simulink model "s7_template"  (R2023a)
settings: Solver=ode4  StartTime=0.0  StopTime=inf  FixedStep=P_sim_dt  RelTol=1e-3
InitFcn:
  | s6_data;
values from neighbouring files (symbols this model uses):
  P_cx_k = 1    [s6_data.m]
  P_p_Bf = 0.7    [p_mad_car.m]
  P_p_Br = 0.7    [p_mad_car.m]
  P_p_Cf = 2    [p_mad_car.m]
  P_p_Cr = 2    [p_mad_car.m]
  P_p_delta_max = 21.58/180*pi    (= 0.37664205258)    [p_mad_car.m]
  P_p_Df = 2    [p_mad_car.m]
  P_p_Dr = 2.5    [p_mad_car.m]
  P_p_Ef = -0.1    [p_mad_car.m]
  P_p_Er = -0.05    [p_mad_car.m]
  P_p_J = 192e-6    (= 0.000192)    [p_mad_car.m]
  P_p_k = 2.51    [p_mad_car.m]
  P_p_kr = 0.344014    [s6_data.m]
  P_p_l = abs(P_p_frontaxle_1 + P_p_rearaxle_1)    [p_mad_car.m]
  P_p_lf = P_p_frontaxle_1    (= 0.05)    [p_mad_car.m]
  P_p_lr = P_p_rearaxle_1    (= 0.049)    [p_mad_car.m]
  P_p_m = 132e-3    (= 0.132)    [p_mad_car.m]
  P_p_T = 316e-3    (= 0.316)    [p_mad_car.m]
  P_p_TA = 0.02    [s6_data.m]
  P_p_Ti = 0.246830    (= 0.24683)    [s6_data.m]
  P_p_Tt = P_p_uTt + P_p_output_Tt    (= 0.1)    [p_mad_car.m]
undefined symbols (not defined in the file or in its folder): DiscIntNeverNeededParam, Display, mad_lib_template, mbc_car_display
settings Model: Creator=hmekiedj  LastModifiedBy=aaron
settings SolverCC: AlgebraicLoopSolver=TrustRegion
settings DataIOCC: ReturnWorkspaceOutputs=off
settings OptimizationCC: BlockReduction=off  DefaultParameterBehavior=Inlined  BufferReuse=off
settings DebuggingCC: SignalInfNanChecking=warning  UnconnectedInputMsg=warning  UnconnectedOutputMsg=warning  UnconnectedLineMsg=warning  ArithmeticOperatorsInVariantConditions=warning
settings ModelReferenceCC: EnableRefExpFcnMdlSchedulingChecks=on
settings SFSimCC: SimUseLocalCustomCode=off  CustomCodeUndefinedFunction=UseInterfaceOnly
settings RTWCC: RTWUseLocalCustomCode=off
settings CodeAppCC: StateflowObjectComments=on

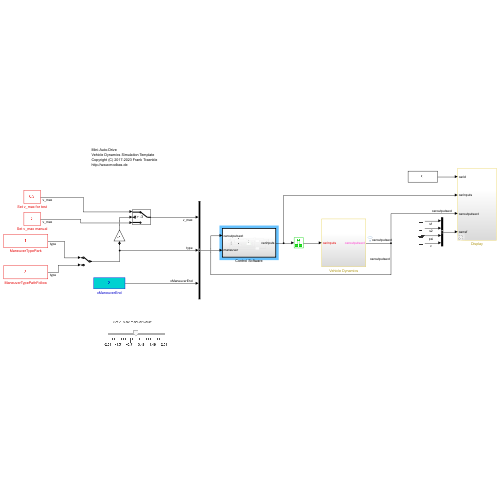
[thumbnail: Simulink's stored preview of the top-level diagram]
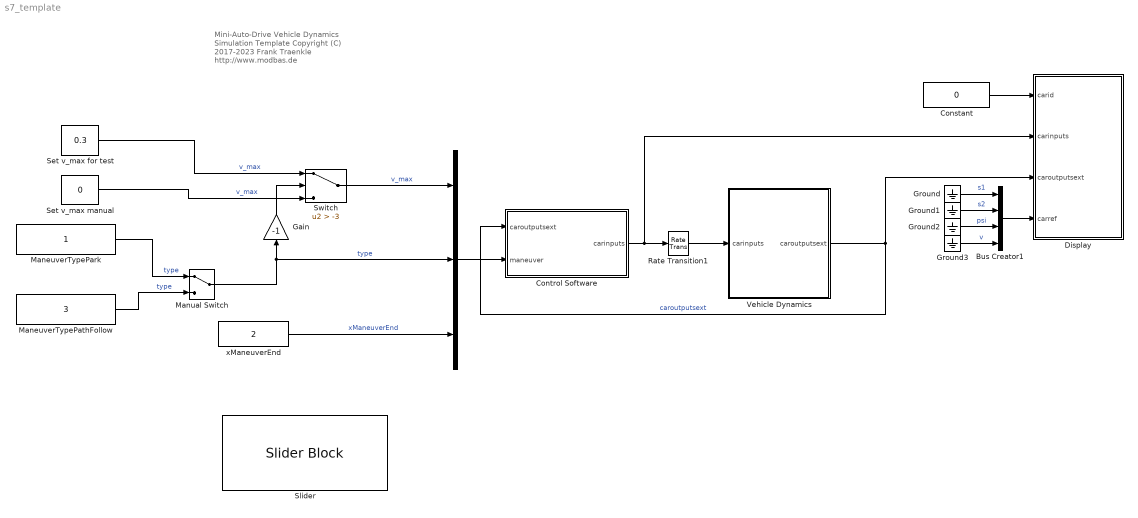
== system s7_template ==
  note: Mini-Auto-Drive
      | Vehicle Dynamics Simulation Template
      | Copyright (C) 2017-2023 Frank Traenkle
      | http://www.modbas.de
  " " : BusCreator  Inputs=3
  Bus Creator1 : BusCreator  Inputs=4
  Constant : Constant  Value=0
  Control Software : Subsystem  TreatAsAtomicUnit=on  SystemSampleTime=P_p_TA
  Display : Subsystem  AncestorBlock=mad_lib_template/Display
      settings: LibrarySourceBlock=mad_lib_template/Display
  Gain : Gain  Gain=-1
  Ground{,1..3} (4 alike) : Ground
  ManeuverTypePark : Constant  SampleTime=-1
  ManeuverTypePathFollow : Constant  Value=3  SampleTime=-1
  Manual Switch : ManualSwitch
  Rate Transition1 : RateTransition
  Set v_max for test : Constant  Value=0.3  SampleTime=-1
  Set v_max manual : Constant  Value=0  SampleTime=-1
  Slider : SliderBlock  ScaleMin=-2.51  ScaleMax=2.51
  Switch : Switch  Criteria=u2 > Threshold  Threshold=-3  SaturateOnIntegerOverflow=off  InputSameDT=off
  Vehicle Dynamics : Subsystem
  xManeuverEnd : Constant  Value=2
  wires:
  Bus Creator1/1 -> Display/4(carref)
  Ground/1 -> Bus Creator1/1  "s1"
  Ground1/1 -> Bus Creator1/2  "s2"
  Ground2/1 -> Bus Creator1/3  "psi"
  Ground3/1 -> Bus Creator1/4  "v"
  Vehicle Dynamics/1(caroutputsext) -> Display/3(caroutputsext), Control Software/1(caroutputsext)  "caroutputsext"
  Rate Transition1/1 -> Vehicle Dynamics/1(carinputs)
  Constant/1 -> Display/1(carid)
  Control Software/1(carinputs) -> Display/2(carinputs), Rate Transition1/1
  " "/1 -> Control Software/2(maneuver)
  xManeuverEnd/1 -> " "/3  "xManeuverEnd"
  ManeuverTypePathFollow/1 -> Manual Switch/2  "type"
  ManeuverTypePark/1 -> Manual Switch/1  "type"
  Manual Switch/1 -> " "/2, Gain/1  "type"
  Switch/1 -> " "/1  "v_max"
  Gain/1 -> Switch/2
  Set v_max for test/1 -> Switch/1  "v_max"
  Set v_max manual/1 -> Switch/3  "v_max"

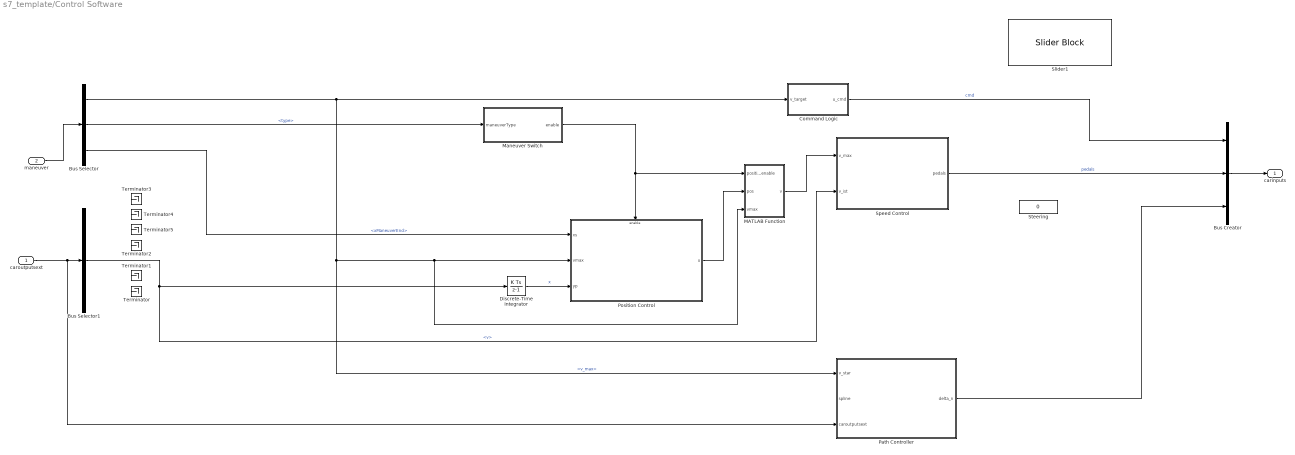
== system s7_template/Control Software ==
  caroutputsext : Inport
  maneuver : Inport  Port=2
  Bus Creator : BusCreator  Inputs=3
  Bus Selector : BusSelector  OutputSignals=v_max,type,xManeuverEnd
  Bus Selector1 : BusSelector  OutputSignals=v
  Command Logic : MATLAB Function  TreatAsAtomicUnit=on
  Discrete-Time Integrator : DiscreteIntegrator  SampleTime=-1  ICPrevOutput=DiscIntNeverNeededParam  ICPrevScaledInput=DiscIntNeverNeededParam
  MATLAB Function : MATLAB Function  TreatAsAtomicUnit=on
  Maneuver Switch : MATLAB Function  TreatAsAtomicUnit=on
  Path Controller : Subsystem
  Position Control : Subsystem
  Slider1 : SliderBlock  LabelPosition=Bottom  ScaleMin=-1  ScaleMax=1
  Speed Control : Subsystem
  Steering : Constant  Value=0  SampleTime=-1
  Terminator{,1..5} (6 alike) : Terminator
  carinputs : Outport
  wires:
  maneuver/1 -> Bus Selector/1
  caroutputsext/1 -> Path Controller/3(caroutputsext), Bus Selector1/1
  Bus Selector1/1 -> Speed Control/2(v_ist), Discrete-Time Integrator/1  "<v>"
  ? -> Terminator/1
  ? -> Terminator1/1
  ? -> Terminator2/1
  ? -> Terminator5/1
  ? -> Terminator4/1
  ? -> Terminator3/1
  Bus Creator/1 -> carinputs/1
  Command Logic/1(u_cmd) -> Bus Creator/1  "cmd"
  Speed Control/1(pedals) -> Bus Creator/2  "pedals"
  Bus Selector/1 -> Path Controller/1(v_star), Position Control/2(vmax), MATLAB Function/3(vmax), Command Logic/1(v_target)  "<v_max>"
  Discrete-Time Integrator/1 -> Position Control/3(yp)  "x"
  Bus Selector/2 -> Maneuver Switch/1(maneuverType)  "<type>"
  Bus Selector/3 -> Position Control/1(xs)  "<xManeuverEnd>"
  Position Control/1(u) -> MATLAB Function/2(pos)
  MATLAB Function/1(v) -> Speed Control/1(v_max)
  Maneuver Switch/1(enable) -> MATLAB Function/1(position_enable), Position Control/Enable
  Path Controller/1(delta_n) -> Bus Creator/3

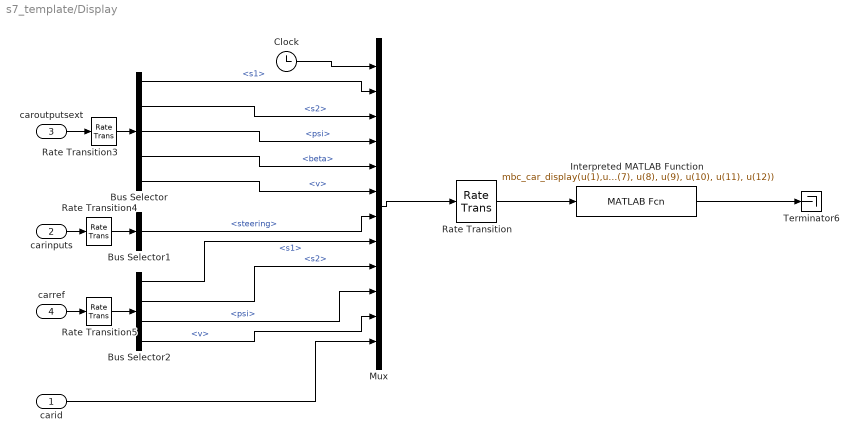
== system s7_template/Display ==
  carid : Inport
  carinputs : Inport  Port=2
  caroutputsext : Inport  Port=3
  carref : Inport  Port=4
  Bus Selector : BusSelector  OutputSignals=s1,s2,psi,beta,v
  Bus Selector1 : BusSelector  OutputSignals=steering
  Bus Selector2 : BusSelector  OutputSignals=s1,s2,psi,v
  Clock : Clock
  Interpreted MATLAB Function : MATLABFcn  MATLABFcn=mbc_car_display(u(1),u(2),u(3),u(4),u(5), u(6), u(7), u(8), u(9), u(10), u(11), u(12))
  Mux : Mux  Inputs=12
  Rate Transition : RateTransition  OutPortSampleTime=P_display_dt
  Rate Transition3 : RateTransition
  Rate Transition4 : RateTransition
  Rate Transition5 : RateTransition
  Terminator6 : Terminator
  wires:
  caroutputsext/1 -> Rate Transition3/1
  Interpreted MATLAB Function/1 -> Terminator6/1
  Mux/1 -> Rate Transition/1
  Rate Transition/1 -> Interpreted MATLAB Function/1
  Clock/1 -> Mux/1
  Bus Selector/1 -> Mux/2  "<s1>"
  Bus Selector/2 -> Mux/3  "<s2>"
  Bus Selector/3 -> Mux/4  "<psi>"
  carinputs/1 -> Rate Transition4/1
  Bus Selector1/1 -> Mux/7  "<steering>"
  Bus Selector/4 -> Mux/5  "<beta>"
  Bus Selector/5 -> Mux/6  "<v>"
  carref/1 -> Rate Transition5/1
  Bus Selector2/4 -> Mux/11  "<v>"
  Bus Selector2/3 -> Mux/10  "<psi>"
  Bus Selector2/2 -> Mux/9  "<s2>"
  Bus Selector2/1 -> Mux/8  "<s1>"
  carid/1 -> Mux/12
  Rate Transition4/1 -> Bus Selector1/1
  Rate Transition3/1 -> Bus Selector/1
  Rate Transition5/1 -> Bus Selector2/1

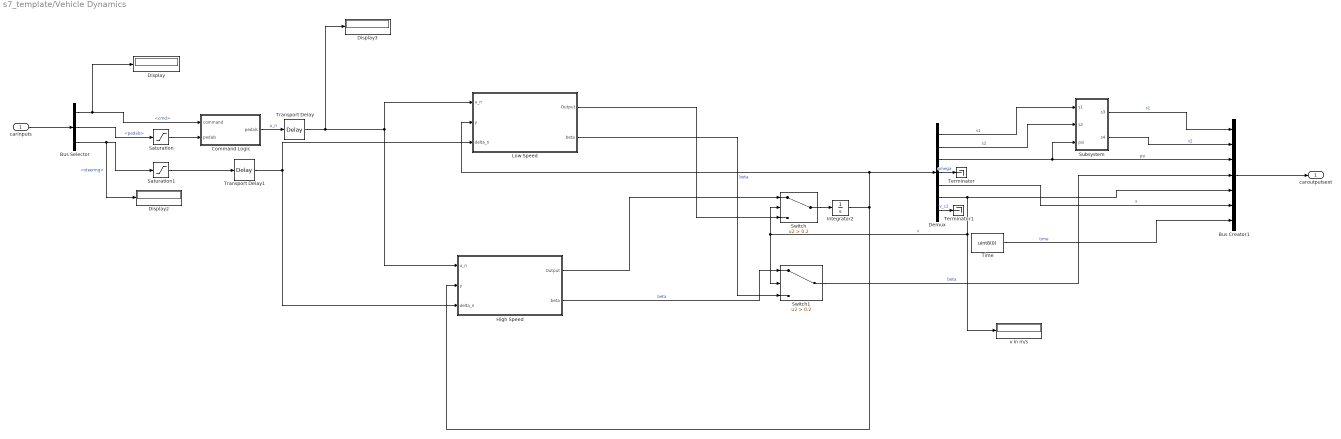
== system s7_template/Vehicle Dynamics ==
  carinputs : Inport
  Bus Creator1 : BusCreator  Inputs=7  OutDataTypeStr=Bus: CAROUTPUTSEXT
  Bus Selector : BusSelector  OutputSignals=cmd,pedals,steering
  Command Logic : MATLAB Function  TreatAsAtomicUnit=on
  Demux : Demux  Outputs=7
  Display : Display
  Display2 : Display
  Display3 : Display
  High Speed : Subsystem
  Integrator2 : Integrator
  Low Speed : Subsystem
  Saturation : Saturate  UpperLimit=1  LowerLimit=-1
  Saturation1 : Saturate  UpperLimit=1  LowerLimit=-1
  Subsystem : Subsystem
  Switch : Switch  Criteria=u2 > Threshold  Threshold=0.2  SaturateOnIntegerOverflow=off  InputSameDT=off
  Switch1 : Switch  Criteria=u2 > Threshold  Threshold=0.2  SaturateOnIntegerOverflow=off  InputSameDT=off
  Terminator : Terminator
  Terminator1 : Terminator
  Time : Constant  Value=uint8(0)
  Transport Delay : TransportDelay  DelayTime=P_p_Tt
  Transport Delay1 : TransportDelay  DelayTime=P_p_Tt
  v in m/s : Display
  caroutputsext : Outport  VectorParamsAs1DForOutWhenUnconnected=off
  wires:
  carinputs/1 -> Bus Selector/1
  Bus Selector/2 -> Saturation/1  "<pedals>"
  Bus Selector/3 -> Saturation1/1, Display2/1  "<steering>"
  Demux/3 -> Subsystem/3(psi), Bus Creator1/3  "psi"
  Bus Creator1/1 -> caroutputsext/1
  Demux/6 -> Switch1/2, Switch/2, v in m/s/1, Bus Creator1/5  "v"
  Time/1 -> Bus Creator1/7  "time"
  Bus Selector/1 -> Display/1, Command Logic/1(command)  "<cmd>"
  Saturation/1 -> Command Logic/2("pedals ")
  Command Logic/1(pedals) -> Transport Delay/1  "u_n"
  Switch/1 -> Integrator2/1
  Transport Delay/1 -> High Speed/1(u_n), Low Speed/1(u_n), Display3/1
  Saturation1/1 -> Transport Delay1/1
  Low Speed/1(Output) -> Switch/3
  Low Speed/2(beta) -> Switch1/3  "beta"
  Switch1/1 -> Bus Creator1/4  "beta"
  Demux/4 -> Terminator/1  "omega"
  High Speed/1(Output) -> Switch/1
  Demux/7 -> Terminator1/1  "v_c2"
  Integrator2/1 -> High Speed/2(y), Low Speed/2(y), Demux/1
  Transport Delay1/1 -> High Speed/3(delta_n), Low Speed/3(delta_n)
  Demux/1 -> Subsystem/1(s1)  "s1"
  Demux/2 -> Subsystem/2(s2)  "s2"
  Subsystem/1(s3) -> Bus Creator1/1  "s1"
  Subsystem/2(s4) -> Bus Creator1/2  "s2"
  Demux/5 -> Bus Creator1/6  "x"
  High Speed/2(beta) -> Switch1/1  "beta"

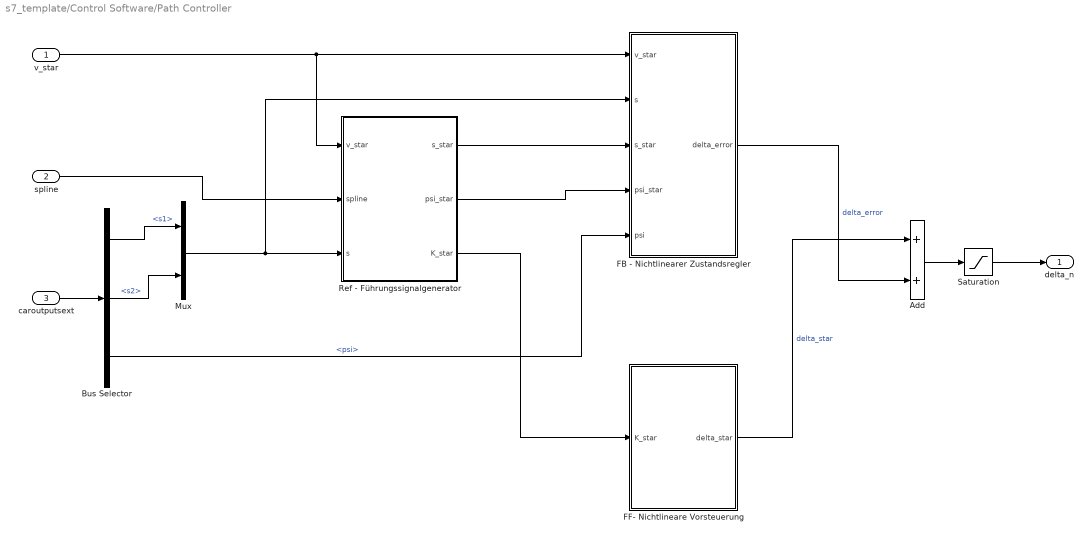
== system s7_template/Control Software/Path Controller ==
  v_star : Inport
  spline : Inport  Port=2
  caroutputsext : Inport  Port=3
  Add : Sum
  Bus Selector : BusSelector  OutputSignals=s1,s2,psi
  FB - Nichtlinearer Zustandsregler : Subsystem
  FF- Nichtlineare Vorsteuerung : Subsystem
  Mux : Mux  Inputs=2
  Ref - Führungssignalgenerator : Subsystem
  Saturation : Saturate  UpperLimit=1  LowerLimit=-1
  delta_n : Outport
  wires:
  FF- Nichtlineare Vorsteuerung/1(delta_star) -> Add/1  "delta_star"
  FB - Nichtlinearer Zustandsregler/1(delta_error) -> Add/2  "delta_error"
  Saturation/1 -> delta_n/1
  Add/1 -> Saturation/1
  v_star/1 -> FB - Nichtlinearer Zustandsregler/1(v_star), Ref - Führungssignalgenerator/1(v_star)
  spline/1 -> Ref - Führungssignalgenerator/2(spline)
  Ref - Führungssignalgenerator/3(K_star) -> FF- Nichtlineare Vorsteuerung/1(K_star)
  Ref - Führungssignalgenerator/2(psi_star) -> FB - Nichtlinearer Zustandsregler/4(psi_star)
  Ref - Führungssignalgenerator/1(s_star) -> FB - Nichtlinearer Zustandsregler/3(s_star)
  Bus Selector/3 -> FB - Nichtlinearer Zustandsregler/5(psi)  "<psi>"
  caroutputsext/1 -> Bus Selector/1
  Bus Selector/1 -> Mux/1  "<s1>"
  Bus Selector/2 -> Mux/2  "<s2>"
  Mux/1 -> Ref - Führungssignalgenerator/3(s), FB - Nichtlinearer Zustandsregler/2(s)

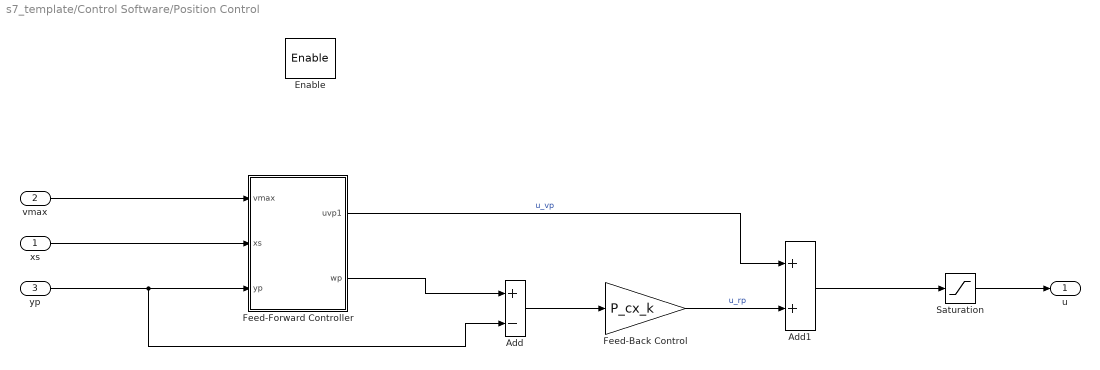
== system s7_template/Control Software/Position Control ==
  xs : Inport
  vmax : Inport  Port=2
  yp : Inport  Port=3
  Enable : EnablePort  StatesWhenEnabling=reset
  Add : Sum  Inputs=+-
  Add1 : Sum
  Feed-Back Control : Gain  Gain=P_cx_k
  Feed-Forward Controller : Subsystem
  Saturation : Saturate  UpperLimit=1  LowerLimit=-1
  u : Outport
  wires:
  Feed-Forward Controller/2(wp) -> Add/1
  Add/1 -> Feed-Back Control/1
  Add1/1 -> Saturation/1
  Saturation/1 -> u/1
  Feed-Back Control/1 -> Add1/2  "u_rp"
  Feed-Forward Controller/1(uvp1) -> Add1/1  "u_vp"
  xs/1 -> Feed-Forward Controller/2(xs)
  vmax/1 -> Feed-Forward Controller/1(vmax)
  yp/1 -> Add/2, Feed-Forward Controller/3(yp)

== system s7_template/Control Software/Speed Control ==
  v_max : Inport
  v_ist : Inport  Port=2
  Add : Sum  Inputs=+-
  Anti-wind-up_ohne_sprung : Subsystem
  Regler : Subsystem
  Saturation1 : Saturate  UpperLimit=1  LowerLimit=-1
  Subsystem : Subsystem  Commented=on
  pedals : Outport
  wires:
  v_max/1 -> Add/1  "v_max"
  v_ist/1 -> Add/2  "v_ist"
  Add/1 -> Regler/1(e)  "e"
  Regler/1(u*) -> Saturation1/1, Anti-wind-up_ohne_sprung/1(u*)  "u*"
  Saturation1/1 -> pedals/1, Anti-wind-up_ohne_sprung/2(u)  "u"
  Anti-wind-up_ohne_sprung/1(windup-error) -> Regler/2(windup-error)

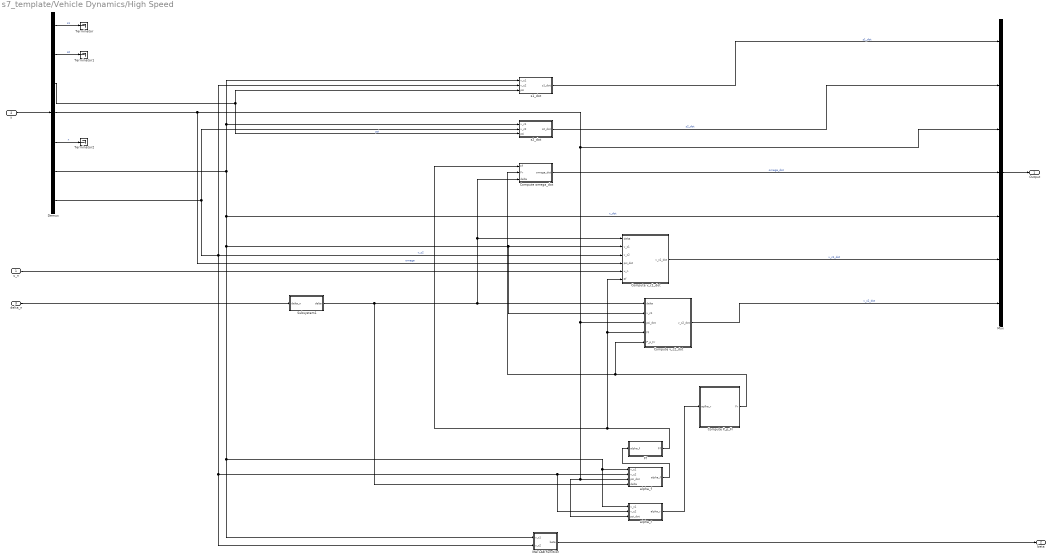
== system s7_template/Vehicle Dynamics/High Speed ==
  u_n : Inport
  y : Inport  Port=2
  delta_n : Inport  Port=3
  Compute P_p_Fr : Subsystem
  Compute omega_dot : Subsystem
  Compute v_c1_dot : Subsystem
  Compute v_c2_dot : Subsystem
  Demux : Demux  Outputs=7
  Ff : Subsystem
  MATLAB Function : MATLAB Function  TreatAsAtomicUnit=on
  Mux : Mux  Inputs=7
  Subsystem1 : Subsystem
  Terminator : Terminator
  Terminator1 : Terminator
  Terminator2 : Terminator
  alpha_f : Subsystem
  alpha_r : Subsystem
  s1_dot : MATLAB Function  TreatAsAtomicUnit=on
  s2_dot : MATLAB Function  TreatAsAtomicUnit=on
  Output : Outport
  beta : Outport  Port=2
  wires:
  Mux/1 -> Output/1
  s1_dot/1(s1_dot) -> Mux/1  "s1_dot"
  Subsystem1/1(delta) -> alpha_f/4(delta), Compute omega_dot/3(delta), Compute v_c1_dot/1(delta), Compute v_c2_dot/1(delta)
  s2_dot/1(s2_dot) -> Mux/2  "s2_dot"
  u_n/1 -> Compute v_c1_dot/5(u_n)
  Demux/1 -> Terminator/1  "s1"
  Demux/2 -> Terminator1/1  "s2"
  Demux/5 -> Terminator2/1  "x"
  Compute v_c1_dot/1(v_c1_dot) -> Mux/6  "v_c1_dot"
  Compute v_c2_dot/1(v_c2_dot) -> Mux/7  "v_c2_dot"
  Demux/7 -> s2_dot/2(v_c2), s1_dot/2(v_c2), Compute v_c1_dot/3(v_c2), alpha_r/2(v_c2), alpha_f/2(v_c2), MATLAB Function/2(v_c2)  "v_c2"
  MATLAB Function/1(beta) -> beta/1
  Compute P_p_Fr/1(Fr) -> Compute omega_dot/2(Fr), Compute v_c2_dot/5(P_p_Fr)
  Ff/1(Ff) -> Compute omega_dot/1(Ff), Compute v_c1_dot/6(Ff), Compute v_c2_dot/4(Ff)
  alpha_f/1(alpha_f) -> Ff/1(alpha_f)
  alpha_r/1(alpha_r) -> Compute P_p_Fr/1(aplha_r)
  delta_n/1 -> Subsystem1/1(delta_n)
  Demux/3 -> s1_dot/3(psi), s2_dot/3(psi)  "psi"
  Demux/4 -> Mux/3, alpha_r/3(psi_dot), alpha_f/3(psi_dot), Compute v_c2_dot/3(psi_dot), Compute v_c1_dot/4(psi_dot)  "omega"
  Compute omega_dot/1(omega_dot) -> Mux/4  "omega_dot"
  y/1 -> Demux/1
  Demux/6 -> Mux/5, alpha_r/1(v_c1), alpha_f/1(v_c1), MATLAB Function/1(v_c1), Compute v_c2_dot/2(v_c1), Compute v_c1_dot/2(v_c1), s2_dot/1(v_c1), s1_dot/1(v_c1)  "x_dot"

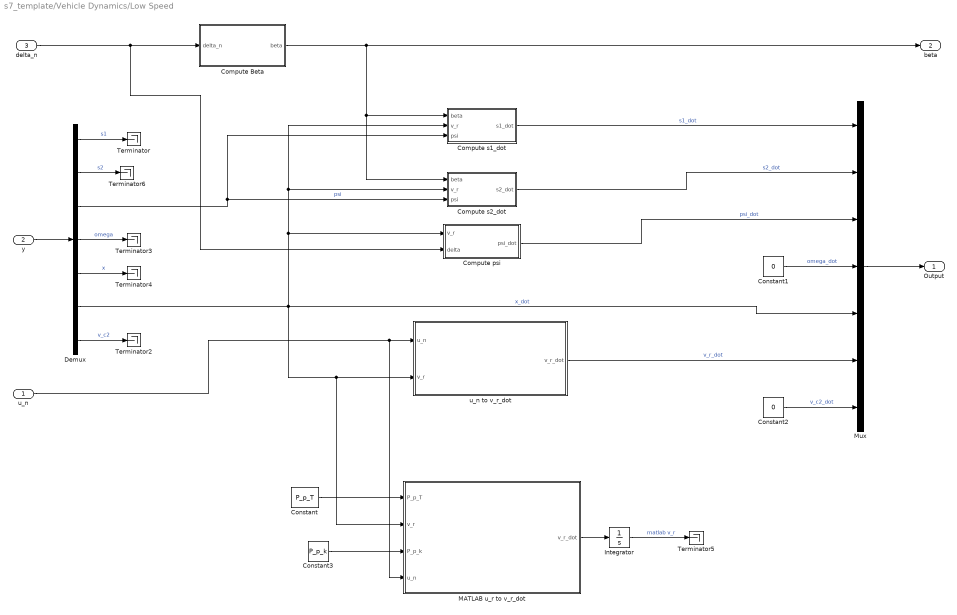
== system s7_template/Vehicle Dynamics/Low Speed ==
  u_n : Inport
  y : Inport  Port=2
  delta_n : Inport  Port=3
  Compute Beta : Subsystem
  Compute psi : Subsystem
  Compute s1_dot : MATLAB Function  TreatAsAtomicUnit=on
  Compute s2_dot : MATLAB Function  TreatAsAtomicUnit=on
  Constant : Constant  Value=P_p_T
  Constant1 : Constant  Value=0
  Constant2 : Constant  Value=0
  Constant3 : Constant  Value=P_p_k
  Demux : Demux  Outputs=7
  Integrator : Integrator
  MATLAB u_r to v_r_dot : MATLAB Function  TreatAsAtomicUnit=on
  Mux : Mux  Inputs=7
  Terminator{,2..6} (6 alike) : Terminator
  u_n to v_r_dot : Subsystem
  Output : Outport
  beta : Outport  Port=2
  wires:
  y/1 -> Demux/1
  Mux/1 -> Output/1
  Demux/3 -> Compute s1_dot/3(psi), Compute s2_dot/3(psi)  "psi"
  delta_n/1 -> Compute psi/2(delta), Compute Beta/1(delta_n)
  Compute s1_dot/1(s1_dot) -> Mux/1  "s1_dot"
  Compute Beta/1(beta) -> Compute s2_dot/1(beta), Compute s1_dot/1(beta), beta/1
  Compute s2_dot/1(s2_dot) -> Mux/2  "s2_dot"
  Compute psi/1(psi_dot) -> Mux/3  "psi_dot"
  Demux/6 -> MATLAB u_r to v_r_dot/2(v_r), u_n to v_r_dot/2(v_r), Mux/5, Compute s1_dot/2(v_r), Compute s2_dot/2(v_r), Compute psi/1(v_r)  "x_dot"
  u_n/1 -> u_n to v_r_dot/1(u_n), MATLAB u_r to v_r_dot/4(u_n)
  Demux/5 -> Terminator4/1  "x"
  Constant1/1 -> Mux/4  "omega_dot"
  Constant2/1 -> Mux/7  "v_c2_dot"
  Demux/4 -> Terminator3/1  "omega"
  Demux/7 -> Terminator2/1  "v_c2"
  Constant/1 -> MATLAB u_r to v_r_dot/1(P_p_T)
  Constant3/1 -> MATLAB u_r to v_r_dot/3(P_p_k)
  MATLAB u_r to v_r_dot/1(v_r_dot) -> Integrator/1
  u_n to v_r_dot/1(v_r_dot) -> Mux/6  "v_r_dot"
  Integrator/1 -> Terminator5/1  "matlab v_r"
  Demux/1 -> Terminator/1  "s1"
  Demux/2 -> Terminator6/1  "s2"

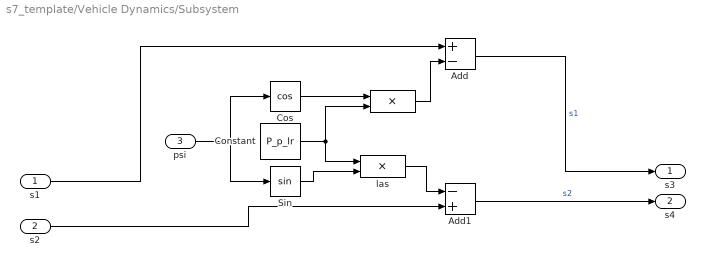
== system s7_template/Vehicle Dynamics/Subsystem ==
  s1 : Inport
  s2 : Inport  Port=2
  psi : Inport  Port=3
  " " : Product
  Add : Sum  Inputs=+-
  Add1 : Sum  Inputs=-+
  Constant : Constant  Value=P_p_lr
  Cos : Trigonometry  Operator=cos
  Sin : Trigonometry
  las : Product
  s3 : Outport
  s4 : Outport  Port=2
  wires:
  Constant/1 -> " "/2, las/1
  Cos/1 -> " "/1
  " "/1 -> Add/2
  psi/1 -> Sin/1, Cos/1
  Sin/1 -> las/2
  las/1 -> Add1/1
  s1/1 -> Add/1
  Add/1 -> s3/1  "s1"
  Add1/1 -> s4/1  "s2"
  s2/1 -> Add1/2

== system s7_template/Control Software/Path Controller/FB - Nichtlinearer Zustandsregler ==
  v_star : Inport
  s : Inport  Port=2
  s_star : Inport  Port=3
  psi_star : Inport  Port=4
  psi : Inport  Port=5
  delta_error : Outport
  wires:
  v_star/1 -> delta_error/1

== system s7_template/Control Software/Path Controller/FF- Nichtlineare Vorsteuerung ==
  K_star : Inport
  delta_star : Outport
  wires:
  K_star/1 -> delta_star/1

== system s7_template/Control Software/Path Controller/Ref - Führungssignalgenerator ==
  v_star : Inport
  spline : Inport  Port=2
  s : Inport  Port=3
  MATLAB Function : MATLAB Function  TreatAsAtomicUnit=on
  s_star : Outport
  psi_star : Outport  Port=2
  K_star : Outport  Port=3
  wires:
  s/1 -> MATLAB Function/2(s)
  spline/1 -> MATLAB Function/1(spline)
  v_star/1 -> MATLAB Function/3(v_star)

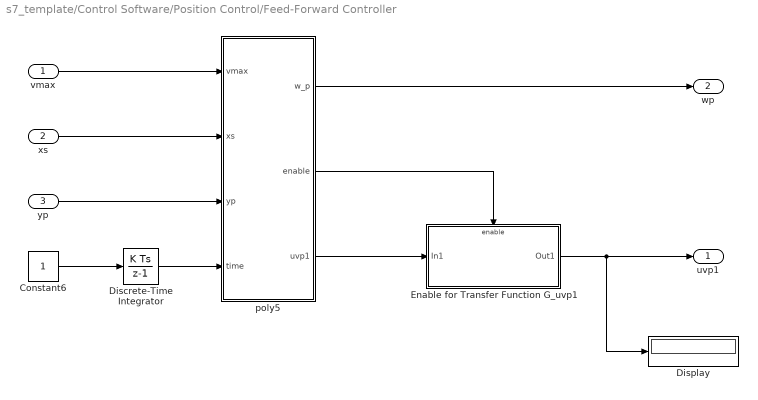
== system s7_template/Control Software/Position Control/Feed-Forward Controller ==
  vmax : Inport
  xs : Inport  Port=2
  yp : Inport  Port=3
  Constant6 : Constant
  Discrete-Time Integrator : DiscreteIntegrator  SampleTime=-1  ICPrevOutput=DiscIntNeverNeededParam  ICPrevScaledInput=DiscIntNeverNeededParam
  Display : Display
  "Enable for Transfer Function G_uvp1 " : Subsystem
  poly5 : MATLAB Function  TreatAsAtomicUnit=on
  uvp1 : Outport
  wp : Outport  Port=2
  wires:
  yp/1 -> poly5/3(yp)
  vmax/1 -> poly5/1(vmax)
  xs/1 -> poly5/2(xs)
  poly5/1(w_p) -> wp/1
  Discrete-Time Integrator/1 -> poly5/4(time)
  Constant6/1 -> Discrete-Time Integrator/1
  poly5/3(uvp1) -> "Enable for Transfer Function G_uvp1 "/1(In1)
  "Enable for Transfer Function G_uvp1 "/1(Out1) -> uvp1/1, Display/1
  poly5/2(enable) -> "Enable for Transfer Function G_uvp1 "/Enable

== system s7_template/Control Software/Speed Control/Anti-wind-up_ohne_sprung ==
  note: Anti-wind-up without hard switch
  u* : Inport
  u : Inport  Port=2
  Gain : Gain  Gain=0.1
  Sum : Sum  Inputs=|-+
  Unit Delay : UnitDelay  SampleTime=-1  HasFrameUpgradeWarning=on
  windup-error : Outport
  wires:
  u*/1 -> Sum/1
  u/1 -> Sum/2
  Sum/1 -> Gain/1
  Gain/1 -> Unit Delay/1
  Unit Delay/1 -> windup-error/1

== system s7_template/Control Software/Speed Control/Regler ==
  e : Inport
  windup-error : Inport  Port=2
  Add : Sum
  Add1 : Sum  Inputs=+++
  Delay : Delay  DelayLength=1  SampleTime=0.02
  Gain : Gain  Gain=P_p_kr
  Gain1 : Gain  Gain=(P_p_kr*P_p_TA) / P_p_Ti
  u* : Outport
  wires:
  Add/1 -> u*/1  "u*"
  Gain/1 -> Add/1  "u_pk"
  e/1 -> Gain/1, Gain1/1
  Gain1/1 -> Add1/2
  Delay/1 -> Add1/1
  Add1/1 -> Delay/1, Add/2  "u_ik"
  windup-error/1 -> Add1/3

== system s7_template/Control Software/Speed Control/Subsystem ==
  u : Inport
  u* : Inport  Port=2
  MATLAB Function : MATLAB Function  TreatAsAtomicUnit=on
  I_condition : Outport
  wires:
  MATLAB Function/1(y) -> I_condition/1
  u/1 -> MATLAB Function/1(u)
  u*/1 -> MATLAB Function/2(u_stern)

== system s7_template/Vehicle Dynamics/High Speed/Compute P_p_Fr ==
  aplha_r : Inport
  Calc_Fr : MATLAB Function  TreatAsAtomicUnit=on
  Constant : Constant  Value=P_p_Br
  Constant1 : Constant  Value=P_p_Cr
  Constant2 : Constant  Value=P_p_Dr
  Constant3 : Constant  Value=P_p_Er
  Fr : Outport
  wires:
  aplha_r/1 -> Calc_Fr/5(alpha_r)
  Constant3/1 -> Calc_Fr/4(P_p_Er)
  Constant2/1 -> Calc_Fr/3(P_p_Dr)
  Constant1/1 -> Calc_Fr/2(P_p_Cr)
  Constant/1 -> Calc_Fr/1(P_p_Br)
  Calc_Fr/1(Fr) -> Fr/1

== system s7_template/Vehicle Dynamics/High Speed/Compute omega_dot ==
  Ff : Inport
  Fr : Inport  Port=2
  delta : Inport  Port=3
  Constant : Constant  Value=P_p_lf
  Constant1 : Constant  Value=P_p_J
  Constant2 : Constant  Value=P_p_lr
  MATLAB Function1 : MATLAB Function  TreatAsAtomicUnit=on
  omega_dot : Outport
  wires:
  MATLAB Function1/1(omega_dot) -> omega_dot/1
  Constant1/1 -> MATLAB Function1/1(P_p_J)
  Ff/1 -> MATLAB Function1/2(Ff)
  Fr/1 -> MATLAB Function1/6(Fr)
  Constant/1 -> MATLAB Function1/3(P_p_lf)
  Constant2/1 -> MATLAB Function1/4(P_p_lr)
  delta/1 -> MATLAB Function1/5(delta)

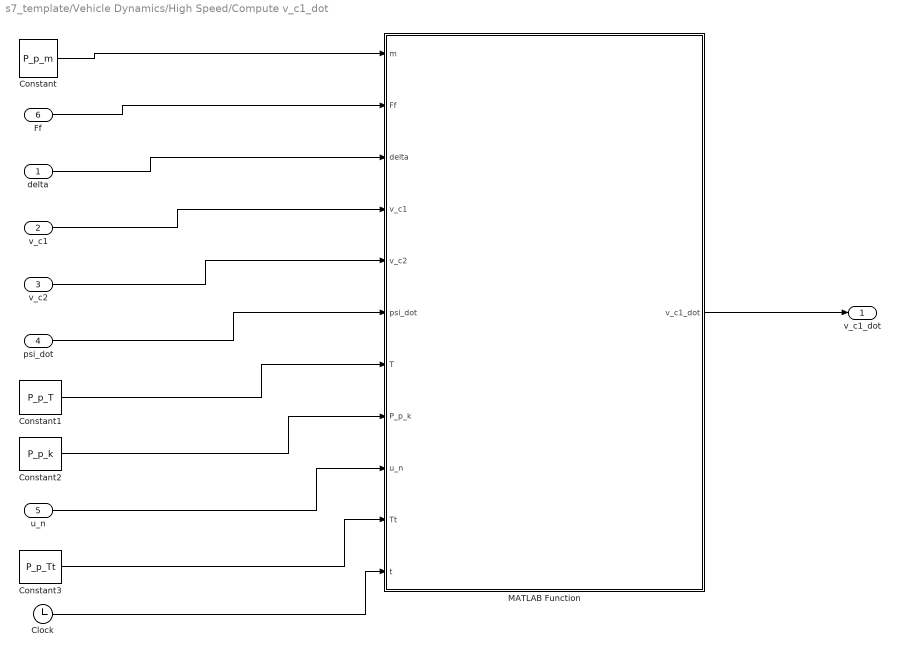
== system s7_template/Vehicle Dynamics/High Speed/Compute v_c1_dot ==
  delta : Inport
  v_c1 : Inport  Port=2
  v_c2 : Inport  Port=3
  psi_dot : Inport  Port=4
  u_n : Inport  Port=5
  Ff : Inport  Port=6
  Clock : Clock
  Constant : Constant  Value=P_p_m
  Constant1 : Constant  Value=P_p_T
  Constant2 : Constant  Value=P_p_k
  Constant3 : Constant  Value=P_p_Tt
  MATLAB Function : MATLAB Function  TreatAsAtomicUnit=on
  v_c1_dot : Outport
  wires:
  MATLAB Function/1(v_c1_dot) -> v_c1_dot/1
  delta/1 -> MATLAB Function/3(delta)
  v_c1/1 -> MATLAB Function/4(v_c1)
  v_c2/1 -> MATLAB Function/5(v_c2)
  psi_dot/1 -> MATLAB Function/6(psi_dot)
  u_n/1 -> MATLAB Function/9(u_n)
  Constant/1 -> MATLAB Function/1(m)
  Ff/1 -> MATLAB Function/2(Ff)
  Constant1/1 -> MATLAB Function/7(T)
  Constant2/1 -> MATLAB Function/8(P_p_k)
  Constant3/1 -> MATLAB Function/10(Tt)
  Clock/1 -> MATLAB Function/11(t)

== system s7_template/Vehicle Dynamics/High Speed/Compute v_c2_dot ==
  delta : Inport
  v_c1 : Inport  Port=2
  psi_dot : Inport  Port=3
  Ff : Inport  Port=4
  P_p_Fr : Inport  Port=5
  Constant : Constant  Value=P_p_m
  MATLAB Function : MATLAB Function  TreatAsAtomicUnit=on
  v_c2_dot : Outport
  wires:
  MATLAB Function/1(v_c2_dot) -> v_c2_dot/1
  delta/1 -> MATLAB Function/4(delta)
  v_c1/1 -> MATLAB Function/5(v_c1)
  P_p_Fr/1 -> MATLAB Function/3(Fr)
  psi_dot/1 -> MATLAB Function/6(psi_dot)
  Constant/1 -> MATLAB Function/1(m)
  Ff/1 -> MATLAB Function/2(Ff)

== system s7_template/Vehicle Dynamics/High Speed/Ff ==
  alpha_f : Inport
  Calc_Ff : MATLAB Function  TreatAsAtomicUnit=on
  Constant : Constant  Value=P_p_Bf
  Constant1 : Constant  Value=P_p_Cf
  Constant2 : Constant  Value=P_p_Df
  Constant3 : Constant  Value=P_p_Ef
  Ff : Outport
  wires:
  alpha_f/1 -> Calc_Ff/5(alpha_f)
  Constant1/1 -> Calc_Ff/2(P_p_Cf)
  Constant/1 -> Calc_Ff/1(P_p_Bf)
  Constant3/1 -> Calc_Ff/4(P_p_Ef)
  Constant2/1 -> Calc_Ff/3(P_p_Df)
  Calc_Ff/1(Ff) -> Ff/1

== system s7_template/Vehicle Dynamics/High Speed/Subsystem1 ==
  delta_n : Inport
  Clock : Clock
  Constant : Constant  Value=P_p_delta_max
  Constant1 : Constant  Value=P_p_Tt
  MATLAB Function : MATLAB Function  TreatAsAtomicUnit=on
  delta : Outport
  wires:
  MATLAB Function/1(delta) -> delta/1
  Clock/1 -> MATLAB Function/3(t)
  Constant1/1 -> MATLAB Function/4(P_p_Tt)
  Constant/1 -> MATLAB Function/2(delta_n)
  delta_n/1 -> MATLAB Function/1(P_p_delta_max)

== system s7_template/Vehicle Dynamics/High Speed/alpha_f ==
  v_c1 : Inport
  v_c2 : Inport  Port=2
  psi_dot : Inport  Port=3
  delta : Inport  Port=4
  Constant : Constant  Value=P_p_lf
  MATLAB Function : MATLAB Function  TreatAsAtomicUnit=on
  alpha_f : Outport
  wires:
  v_c1/1 -> MATLAB Function/1(v_c1)
  v_c2/1 -> MATLAB Function/2(v_c2)
  Constant/1 -> MATLAB Function/3(P_p_lf)
  psi_dot/1 -> MATLAB Function/4(psi_dot)
  MATLAB Function/1(alpha_f) -> alpha_f/1
  delta/1 -> MATLAB Function/5(delta)

== system s7_template/Vehicle Dynamics/High Speed/alpha_r ==
  v_c1 : Inport
  v_c2 : Inport  Port=2
  psi_dot : Inport  Port=3
  Constant : Constant  Value=P_p_lr
  MATLAB Function : MATLAB Function  TreatAsAtomicUnit=on
  alpha_r : Outport
  wires:
  v_c1/1 -> MATLAB Function/1(v_c1)
  v_c2/1 -> MATLAB Function/2(v_c2)
  Constant/1 -> MATLAB Function/3(P_p_lr)
  psi_dot/1 -> MATLAB Function/4(psi_dot)
  MATLAB Function/1(alpha_r) -> alpha_r/1

== system s7_template/Vehicle Dynamics/Low Speed/Compute Beta ==
  delta_n : Inport
  Clock : Clock
  Constant1 : Constant  Value=P_p_l
  Constant2 : Constant  Value=P_p_lr
  Constant3 : Constant  Value=P_p_delta_max
  Constant4 : Constant  Value=P_p_Tt
  MATLAB Function1 : MATLAB Function  TreatAsAtomicUnit=on
  beta : Outport
  wires:
  Constant3/1 -> MATLAB Function1/4(delta_max)
  Constant1/1 -> MATLAB Function1/2(P_p_l)
  Constant4/1 -> MATLAB Function1/6(Tt)
  MATLAB Function1/1(beta) -> beta/1
  Constant2/1 -> MATLAB Function1/1(a)
  Clock/1 -> MATLAB Function1/5(t)
  delta_n/1 -> MATLAB Function1/3(delta_n)

== system s7_template/Vehicle Dynamics/Low Speed/Compute psi ==
  v_r : Inport
  delta : Inport  Port=2
  Clock : Clock
  Constant1 : Constant  Value=P_p_l
  Constant3 : Constant  Value=P_p_delta_max
  Constant4 : Constant  Value=P_p_Tt
  MATLAB Function1 : MATLAB Function  TreatAsAtomicUnit=on
  psi_dot : Outport
  wires:
  Constant3/1 -> MATLAB Function1/4(delta_max)
  Constant1/1 -> MATLAB Function1/2(l)
  Constant4/1 -> MATLAB Function1/6(Tt)
  MATLAB Function1/1(psi_dot) -> psi_dot/1
  v_r/1 -> MATLAB Function1/1(v_r)
  Clock/1 -> MATLAB Function1/5(t)
  delta/1 -> MATLAB Function1/3(delta)

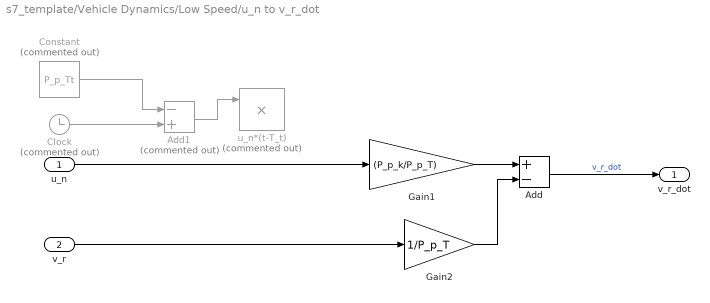
== system s7_template/Vehicle Dynamics/Low Speed/u_n to v_r_dot ==
  u_n : Inport
  v_r : Inport  Port=2
  Add : Sum  Inputs=+-
  Add1 : Sum  Commented=on  Inputs=-+
  Clock : Clock  Commented=on
  Constant : Constant  Commented=on  Value=P_p_Tt
  Gain1 : Gain  Gain=(P_p_k/P_p_T)
  Gain2 : Gain  Gain=1/P_p_T
  u_n*(t-T_t) : Product  Commented=on
  v_r_dot : Outport
  wires:
  Gain2/1 -> Add/2
  Clock/1 -> Add1/2
  u_n/1 -> Gain1/1
  Add1/1 -> u_n*(t-T_t)/1
  Constant/1 -> Add1/1
  Gain1/1 -> Add/1
  Add/1 -> v_r_dot/1  "v_r_dot"
  v_r/1 -> Gain2/1

== system s7_template/Control Software/Position Control/Feed-Forward Controller/Enable for Transfer Function G_uvp1  ==
  In1 : Inport
  Enable : EnablePort
  Discrete Transfer Fcn : DiscreteTransferFcn  Numerator=[2 -2]  Denominator=[(2*P_p_Ti+P_p_T) (P_p_T-2*P_p_Ti)]
  Out1 : Outport
  wires:
  Discrete Transfer Fcn/1 -> Out1/1
  In1/1 -> Discrete Transfer Fcn/1

== matlab function s7_template/Vehicle Dynamics/Low Speed/Compute psi/MATLAB Function1 ==
  data: v_r input; psi_dot output; l input; delta input; delta_max input; t input; Tt input
function psi_dot = fcn(v_r, l, delta, delta_max, t, Tt)

% psi = (v_r/l) * tan(delta_max * delta * (t - Tt) );
psi_dot = (v_r/l) * tan(delta_max * delta);

== matlab function s7_template/Vehicle Dynamics/High Speed/Compute v_c1_dot/MATLAB Function ==
  data: m input; v_c1_dot output; Ff input; delta input; v_c1 input; v_c2 input; psi_dot input; T input; P_p_k input; u_n input; Tt input; t input
function v_c1_dot = fcn(m, Ff, delta, v_c1, v_c2, psi_dot, T, P_p_k, u_n, Tt, t)

% v_c1_dot = (1/m) * (-Ff * sin(delta) + m * v_c2 * psi_dot) ...
%                     - 1/T * v_c1 ...
%                     + (P_p_k/T) * u_n * (t - Tt);


v_c1_dot = (1/m) * (-Ff * sin(delta) + m * v_c2 * psi_dot) ...
                    - 1/T * v_c1 ...
                    + (P_p_k/T) * u_n;

== matlab function s7_template/Vehicle Dynamics/High Speed/Compute v_c2_dot/MATLAB Function ==
  data: m input; v_c2_dot output; Ff input; Fr input; delta input; v_c1 input; psi_dot input
function v_c2_dot = fcn(m, Ff, Fr, delta, v_c1, psi_dot)

v_c2_dot = (1/m) * (Ff * cos(delta) + Fr - m * v_c1 * psi_dot);

== matlab function s7_template/Vehicle Dynamics/High Speed/Compute P_p_Fr/Calc_Fr ==
  data: P_p_Br input; Fr output; P_p_Cr input; P_p_Dr input; P_p_Er input; alpha_r input
function Fr = fcn(P_p_Br, P_p_Cr, P_p_Dr, P_p_Er, alpha_r)

Fr = P_p_Dr * sin(P_p_Cr * atan(P_p_Br * (1 - P_p_Er) * alpha_r ...
    - P_p_Er * atan(P_p_Br * alpha_r)));

== matlab function s7_template/Vehicle Dynamics/High Speed/Ff/Calc_Ff ==
  data: P_p_Bf input; Ff output; P_p_Cf input; P_p_Df input; P_p_Ef input; alpha_f input
function Ff = fcn(P_p_Bf, P_p_Cf, P_p_Df, P_p_Ef, alpha_f)

Ff = P_p_Df * sin(P_p_Cf * atan(P_p_Bf * (1 - P_p_Ef) * alpha_f ...
    - P_p_Ef * atan(P_p_Bf * alpha_f)));

== matlab function s7_template/Vehicle Dynamics/High Speed/alpha_r/MATLAB Function ==
  data: v_c1 input; alpha_r output; v_c2 input; P_p_lr input; psi_dot input
function alpha_r = fcn(v_c1, v_c2, P_p_lr, psi_dot)

if(v_c1 > 0)
    % we will use this equvaltion if the vilocity v_c1 is above 0 (v_c1 > 0)
    alpha_r = -atan((v_c2 - P_p_lr * psi_dot) / v_c1);
elseif (v_c1 < 0)
    % we will use this equvaltion if the vilocity v_c1 is below 0 (v_c1 < 0)
    alpha_r = atan((v_c2 - P_p_lr * psi_dot) / v_c1);
else
    alpha_r = 0;
end

== matlab function s7_template/Vehicle Dynamics/High Speed/Subsystem1/MATLAB Function ==
  data: P_p_delta_max input; delta output; delta_n input; t input; P_p_Tt input
function delta = fcn(P_p_delta_max, delta_n, t, P_p_Tt)

% delta = P_p_delta_max * delta_n*(t-P_p_Tt);
delta = P_p_delta_max * delta_n;

== matlab function s7_template/Vehicle Dynamics/Low Speed/MATLAB u_r to v_r_dot ==
  data: P_p_T input; v_r_dot output; v_r input; P_p_k input; u_n input
function v_r_dot = fcn(P_p_T, v_r, P_p_k, u_n)

v_r_dot = (-1/P_p_T) * v_r + (P_p_k/P_p_T) * u_n;

== matlab function s7_template/Control Software/Speed Control/Subsystem/MATLAB Function ==
  data: u input; y output; u_stern input
function y = fcn(u, u_stern )


if(u ~= u_stern)
    y = 1;
else
    y = 0;
end

== matlab function s7_template/Vehicle Dynamics/High Speed/alpha_f/MATLAB Function ==
  data: v_c1 input; alpha_f output; v_c2 input; P_p_lf input; psi_dot input; delta input
function alpha_f = fcn(v_c1, v_c2, P_p_lf, psi_dot, delta)

if (v_c1 > 0)
    % we will use this equvaltion if the vilocity v_c1 is above 0 (v_c1 > 0)
    alpha_f = -atan((v_c2 + P_p_lf * psi_dot) / v_c1) + delta;
elseif (v_c1 < 0)
    % we will use this equvaltion if the vilocity v_c1 is below 0 (v_c1 < 0)
    alpha_f = atan((v_c2 + P_p_lf * psi_dot) / v_c1) - delta;
else
    alpha_f = 0;
end

== matlab function s7_template/Control Software/Command Logic ==
  data: v_target input; u_cmd output
function u_cmd = fcn(v_target)

    if v_target >= 0
        u_cmd = uint8(1);   % "CarInputsCmdForward"
    else
        u_cmd = uint8(2);   % "CarInputsCmdReverse"
    end
end

== matlab function s7_template/Control Software/Position Control/Feed-Forward Controller/poly5 ==
  data: vmax input; w_p output; enable output; xs input; yp input; uvp1 output; time input; P_p_Ti parameter; P_p_kr parameter; P_p_k parameter; P_p_T parameter; P_p_Tt parameter
function [w_p, enable, uvp1]= fcn(vmax, xs, yp, time, P_p_Ti, P_p_kr, P_p_k, P_p_T, P_p_Tt)
persistent c cff te x0;

% erster Iterationsschritt: x0 mit Rückführung initialisieren, 
% Koeffizienten undte berechnen
if isempty(c)
    x0 = yp;

    [c, te] = cd_refpoly_vmax(vmax, x0, xs);
    %te = te + time
    cff = cd_refpoly_ff(c, P_p_k, P_p_T, P_p_Tt, P_p_kr, P_p_Ti);
end

if time >= te     % fertig
    enable = false;
    % Erzeugung des Polynoms w_p aus den Koeffizienten
    w_p = polyval(c, te);
    % Berechnung von uvp1 durch Verwendung der cd_refpoly_ff.m Funktion
    uvp1 = polyval(cff, te);
else
    enable = true;
    w_p = polyval(c, time);
    uvp1 = polyval(cff, time);
end

== matlab function s7_template/Control Software/Maneuver Switch ==
  data: maneuverType input; enable output
function enable  = maneuverSwitch(maneuverType)

if maneuverType == 1        % Park Maneuver
    enable = 1;
elseif maneuverType == 3    % Path Following
    enable = -1;
else
    enable = 0;
    fprintf("Error occcured in maneuverSwitch - no valid manuever");
end

== matlab function s7_template/Control Software/MATLAB Function ==
  data: position_enable input; v output; pos input; vmax input
function v = fcn(position_enable, pos, vmax)

if position_enable == 1
    v = pos;
else
    v = vmax;
end

== matlab function s7_template/Control Software/Path Controller/Ref - Führungssignalgenerator/MATLAB Function ==
  data: spline input; x_star output; s input; v_star input; P_p_Tt input
function x_star = fcn(spline, s, v_star, P_p_Tt)

breakslen = length(spline.points(1,:));
coeffs = spline.pp;

% Check if the last point's x and y coordinates are equal to the first point's x and y coordinates
isCircular = isequal(p.points(2:3, 1), p.points(2:3, end));

[w, widx] = mbc_spline_get_reference(s , breakslen, spline.points, ...
coeffs, isCircular, v_star, P_p_Tt);

x_star = w(1);

x_dach = x_star + v_star * P_p_Tt;

== matlab function s7_template/Vehicle Dynamics/Command Logic ==
  data: command input; pedals input; pedals output
function pedals = fcn(command, pedals)
    switch command
        case 0      % CarInputsCmdHalt
            pedals = 0;
        case 1  % CarInputsCmdForward 
            if (pedals < 0)
                pedals = 0;
            end
        case 2  % CarInputsCmdReverse 
            if (pedals > 0)
                pedals = 0;
            end
     end
end

== matlab function s7_template/Vehicle Dynamics/High Speed/MATLAB Function ==
  data: v_c1 input; beta output; v_c2 input
function beta = fcn(v_c1, v_c2)

beta = atan2(v_c2, v_c1);

== matlab function s7_template/Vehicle Dynamics/High Speed/Compute omega_dot/MATLAB Function1 ==
  data: P_p_J input; omega_dot output; Ff input; P_p_lf input; P_p_lr input; delta input; Fr input
function omega_dot = fcn(P_p_J, Ff, P_p_lf, P_p_lr, delta, Fr)

omega_dot = (1/P_p_J) * (Ff * P_p_lf * cos(delta) - Fr * P_p_lr);

== matlab function s7_template/Vehicle Dynamics/Low Speed/Compute Beta/MATLAB Function1 ==
  data: a input; beta output; P_p_l input; delta_n input; delta_max input; t input; Tt input
function beta = fcn(a, P_p_l, delta_n, delta_max, t, Tt)

% beta = atan((a/l) * tan(delta_max*delta_n*(t - Tt) )  );
beta = atan( (a/P_p_l) * tan(delta_max * delta_n)  );

== matlab function s7_template/Vehicle Dynamics/High Speed/s2_dot ==
  data: v_c1 input; v_c2 input; s2_dot output; psi input
function s2_dot = fcn(v_c1, v_c2, psi)

s2_dot = v_c1 * sin(psi) + v_c2 * cos(psi);

== matlab function s7_template/Vehicle Dynamics/High Speed/s1_dot ==
  data: v_c1 input; v_c2 input; s1_dot output; psi input
function s1_dot = fcn(v_c1, v_c2, psi)

s1_dot = v_c1 * cos(psi) - v_c2 * sin(psi);

== matlab function s7_template/Vehicle Dynamics/Low Speed/Compute s2_dot ==
  data: beta input; v_r input; s2_dot output; psi input
function s2_dot = fcn(beta, v_r, psi)

s2_dot = (v_r/cos(beta)) * sin(psi + beta);

== matlab function s7_template/Vehicle Dynamics/Low Speed/Compute s1_dot ==
  data: beta input; v_r input; s1_dot output; psi input
function s1_dot = fcn(beta,v_r, psi)

s1_dot =  (v_r/cos(beta))  * cos(psi + beta);
